simulink subsystem "MotorVorsteuerung"  (R2020a)
settings: Solver=VariableStepAuto  StartTime=0.0  StopTime=10.0  RelTol=1e-3
model mask{MotorGain=0, Umax=0}
  mask prompts: MotorGain "Static Motor Gain"; Umax "Begrenzung Umax"
settings Model: Creator=Tobias  LastModifiedBy=Tobias

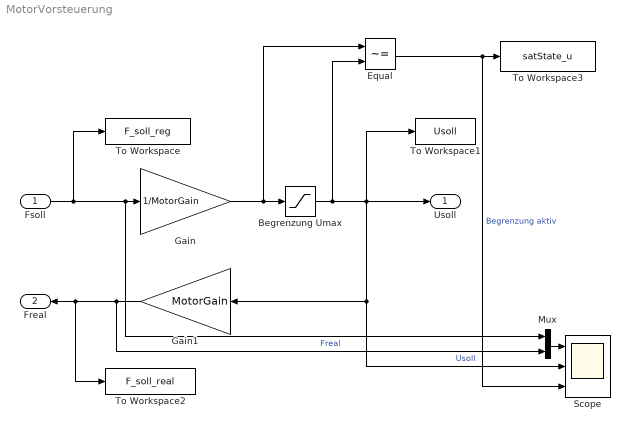
== system MotorVorsteuerung ==
  Fsoll : Inport
  Begrenzung Umax : Saturate  UpperLimit=Umax  LowerLimit=-Umax  ZeroCross=off
  Equal : RelationalOperator  Operator=~=  OutDataTypeStr=boolean  ZeroCross=off  RndMeth=Simplest
  Gain : Gain  Gain=1/MotorGain
  Gain1 : Gain  Gain=MotorGain
  Mux : Mux  Inputs=2
  Scope : Scope  NumInputPorts=3
  To Workspace : ToWorkspace  VariableName=F_soll_reg  SaveFormat=Timeseries  SampleTime=-1
  To Workspace1 : ToWorkspace  VariableName=Usoll  SaveFormat=Timeseries  SampleTime=-1
  To Workspace2 : ToWorkspace  VariableName=F_soll_real  SaveFormat=Timeseries  SampleTime=-1
  To Workspace3 : ToWorkspace  VariableName=satState_u  SaveFormat=Timeseries  SampleTime=-1
  Usoll : Outport
  Freal : Outport  Port=2
  wires:
  Gain/1 -> Begrenzung Umax/1, Equal/1
  Fsoll/1 -> To Workspace/1, Gain/1, Mux/1
  Begrenzung Umax/1 -> To Workspace1/1, Usoll/1, Gain1/1, Scope/2, Equal/2  "Usoll"
  Gain1/1 -> Freal/1, To Workspace2/1, Mux/2  "Freal"
  Equal/1 -> To Workspace3/1, Scope/3  "Begrenzung aktiv"
  Mux/1 -> Scope/1
